simulink model "observer"  (R2022a)
settings: Solver=VariableStepAuto  StartTime=0.0  StopTime=20  RelTol=1e-3
values from neighbouring files (symbols this model uses):
  Ad = sysd.a    [notes.m]
  Bmod = [Bd(1) L(1) ... (first row only)    [notes.m]
  Cd = sysd.c    [notes.m]
  Dd = [0 0 ... (first row only)    [notes.m]
  J = 5.87E-6    (= 5.87e-06)    [notes.m]
  kb = kt    (= 0.0057)    [notes.m]
  kt = 0.0057    [notes.m]
  kv = 2E-6    (= 2e-06)    [notes.m]
  Lm = 300E-6    (= 0.0003)    [notes.m]
  Rm = 2.4    [notes.m]
  Ts = 50E-6    (= 5e-05)    [notes.m]
libraries: simulink x2
settings Model: Creator=Brian  LastModifiedBy=Admin
settings DebuggingCC: UnconnectedInputMsg=warning  UnconnectedOutputMsg=warning  UnconnectedLineMsg=warning
settings RTWCC: DLArmComputeVersion=19.05

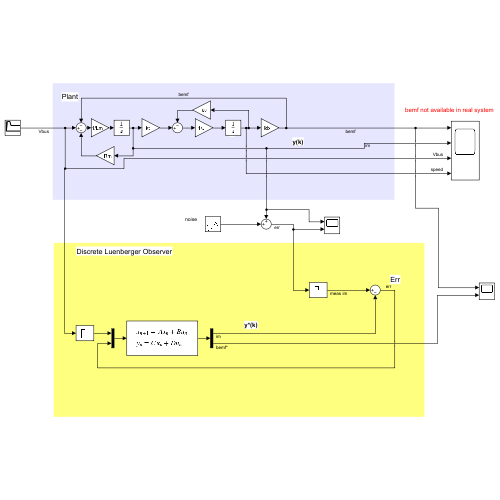
[thumbnail: Simulink's stored preview of the top-level diagram]
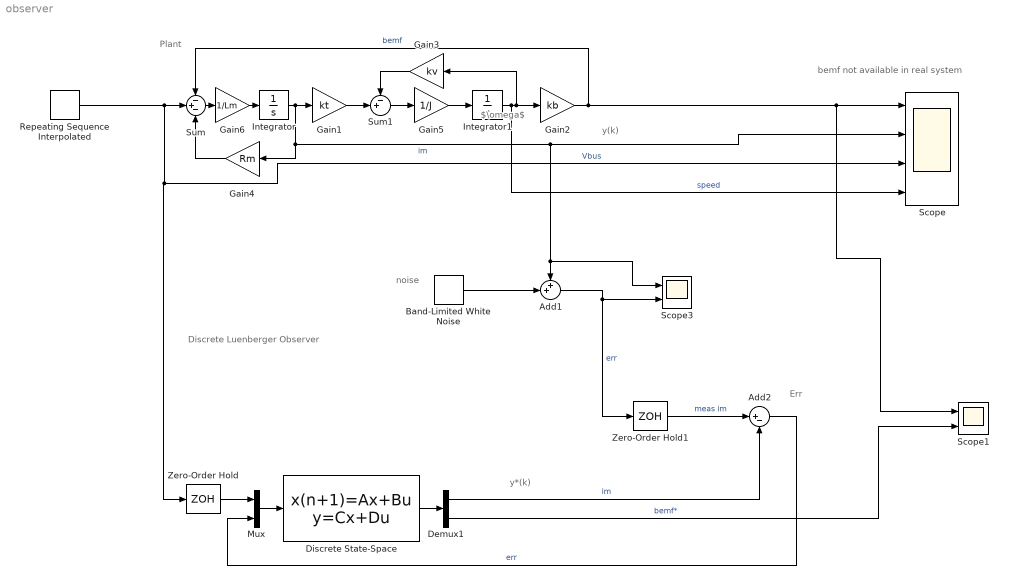
== system observer ==
  note: noise
  note: $\omega$
  note: y(k)
  note: bemf not available in real system
  note: Err
  note: Discrete Luenberger Observer
  note: Plant
  note: y*(k)
  Add1 : Sum  Inputs=++|
  Add2 : Sum  Inputs=|+-
  Band-Limited White Noise : simulink/Sources/Band-Limited White Noise  Cov=2E-6  Ts=Ts  seed=[23341]
  Demux1 : Demux  Outputs=2
  Discrete State-Space : DiscreteStateSpace  A=Ad  B=Bmod  C=Cd  D=Dd  SampleTime=Ts
  Gain1 : Gain  Gain=kt
  Gain2 : Gain  Gain=kb
  Gain3 : Gain  Gain=kv
  Gain4 : Gain  Gain=Rm
  Gain5 : Gain  Gain=1/J
  Gain6 : Gain  Gain=1/Lm
  Integrator : Integrator
  Integrator1 : Integrator
  Mux : Mux  Inputs=2
  Repeating Sequence Interpolated : simulink/Sources/Repeating Sequence Interpolated  OutValues=[0 5 5 3 3].'  TimeValues=[0 2 5 7 20].'  LookUpMeth=Interpolation-Use End Values  tsamp=50E-6  OutMin=[]  OutMax=[]  OutDataTypeStr=double  OutputDataTypeScalingMode=double  OutDataType=fixdt(0,8)  OutScaling=2^-10
  Scope : Scope  NumInputPorts=4
  Scope1 : Scope  NumInputPorts=2
  Scope3 : Scope  NumInputPorts=2
  Sum : Sum  Inputs=-+-
  Sum1 : Sum  Inputs=-+|
  Zero-Order Hold : ZeroOrderHold  SampleTime=Ts
  Zero-Order Hold1 : ZeroOrderHold  SampleTime=Ts
  wires:
  Repeating Sequence Interpolated/1 -> Sum/2, Zero-Order Hold/1, Scope/3  "Vbus"
  Zero-Order Hold1/1 -> Add2/1  "meas im"
  Demux1/1 -> Add2/2  "im"
  Discrete State-Space/1 -> Demux1/1
  Add2/1 -> Mux/2  "err"
  Mux/1 -> Discrete State-Space/1
  Zero-Order Hold/1 -> Mux/1
  Integrator/1 -> Gain1/1, Gain4/1, Scope3/1, Add1/1, Scope/2  "im"
  Integrator1/1 -> Gain3/1, Gain2/1, Scope/4  "speed"
  Gain2/1 -> Sum/1, Scope/1, Scope1/1  "bemf"
  Gain1/1 -> Sum1/2
  Gain3/1 -> Sum1/1
  Gain4/1 -> Sum/3
  Sum1/1 -> Gain5/1
  Gain5/1 -> Integrator1/1
  Sum/1 -> Gain6/1
  Gain6/1 -> Integrator/1
  Add1/1 -> Zero-Order Hold1/1, Scope3/2  "err"
  Band-Limited White Noise/1 -> Add1/2
  Demux1/2 -> Scope1/2  "bemf*"
